simulink model "Distribution_vAggregate"  (Simulink 7.9)
settings: Solver=VariableStepDiscrete  StartTime=0.0  StopTime=1000  RelTol=1e-3
libraries: simeventslib x23
(part 3 of 4)

== system Distribution_vAggregate/Transportation_Channel_41 ==
  note: RESOURCE1 OUTBOUND
      | RESOURCE2 INBOUND
  note: RESOURCE1 INBOUND
      | RESOURCE2 OUTBOUND
  Enabled Gate : EnabledGate
  Enabled Gate1 : EnabledGate
  FIFO Queue : FIFOQueue  Capacity=inf  StatNumberInBlock=on
      settings: OutputPortMap=o1
  FIFO Queue1 : FIFOQueue  Capacity=inf  StatNumberInBlock=on
      settings: OutputPortMap=o1
  Inbound_Process_1 : InfiniteServer  ServiceTimeFrom=Signal port t  ServiceTime=(76.7)/30  StatNumberDeparted=on  StatNumberInBlock=on
      settings: OutputPortMap=o0,o1
  Inbound_Process_2 : InfiniteServer  ServiceTimeFrom=Signal port t  ServiceTime=(76.7)/30  StatNumberDeparted=on  StatNumberInBlock=on
      settings: OutputPortMap=o0,o1
  Inbound_Release_1 : SingleServer  ServiceTime=0  StatNumberInBlock=on
      settings: OutputPortMap=o1
  Inbound_Release_2 : SingleServer  ServiceTime=0  StatNumberInBlock=on
      settings: OutputPortMap=o1
  Infinite Server : InfiniteServer  ServiceTimeFrom=Signal port t  ServiceTime=(76.7)/30
  Infinite Server1 : InfiniteServer  ServiceTimeFrom=Signal port t  ServiceTime=(76.7)/30
  Mux : Mux  Inputs=3
  Outbound_Process_1 : InfiniteServer  ServiceTimeFrom=Signal port t  ServiceTime=(76.7)/30  StatNumberInBlock=on
      settings: OutputPortMap=o1
  Outbound_Process_2 : InfiniteServer  ServiceTimeFrom=Signal port t  ServiceTime=(76.7)/30  StatNumberInBlock=on
      settings: OutputPortMap=o1
  Outbound_Release_1 : SingleServer  ServiceTime=0  StatNumberInBlock=on
      settings: OutputPortMap=o1
  Outbound_Release_2 : SingleServer  ServiceTime=0  StatNumberInBlock=on
      settings: OutputPortMap=o1
  Sum{,1..2,4} (4 alike) : Sum  Inputs=|++
  Sum3 : Sum  Inputs=|++++
  TC_Status : simeventslib/SimEvents Sinks/Discrete Event Signal to Workspace  VariableName=Transportation_Channel_41_Status  SaveFormat=Structure With Time  isMonitorOnly=off  isRecordIC=off
  Timed to Event Signal : TimedToEventSignal
  TravelTime : Constant  Value=95.8472/30
  IN_Shipment_1 : PMIOPort  Port=1  Side=Left
  OUT_Shipment_1 : PMIOPort  Port=2  Side=Right
  IN_Resource_1 : PMIOPort  Port=3  Side=Left
  OUT_Resource_1 : PMIOPort  Port=4  Side=Right
  IN_Shipment_2 : PMIOPort  Port=5  Side=Left
  OUT_Shipment_2 : PMIOPort  Port=6  Side=Right
  IN_Resource_2 : PMIOPort  Port=7  Side=Left
  OUT_Resource_2 : PMIOPort  Port=8  Side=Right
  tag scope: Transportation_Channel_41_Status=global
  wires:
  Sum4/1 -> Mux/3
  Inbound_Process_2/1 -> Sum4/2
  Inbound_Process_1/1 -> Sum4/1
  Inbound_Process_2/2 -> Sum3/4
  Outbound_Process_2/1 -> Sum3/3
  Inbound_Process_1/2 -> Sum3/2
  Outbound_Process_1/1 -> Sum3/1
  Sum3/1 -> Mux/2
  Sum/1 -> Mux/1
  Mux/1 -> TC_Status/1, [Transportation_Channel_41_Status]
  Inbound_Release_2/1 -> Sum2/2
  Outbound_Release_1/1 -> Sum2/1
  Sum2/1 -> Enabled Gate/1
  Inbound_Release_1/1 -> Sum1/1
  Outbound_Release_2/1 -> Sum1/2
  Sum1/1 -> Enabled Gate1/1
  Timed to Event Signal/1 -> Infinite Server/1, Inbound_Process_2/1, Inbound_Process_1/1, Infinite Server1/1, Outbound_Process_2/1, Outbound_Process_1/1
  TravelTime/1 -> Timed to Event Signal/1
  FIFO Queue/1 -> Sum/1
  FIFO Queue1/1 -> Sum/2
  connections:
  Inbound_Process_1/RConn1 -- OUT_Resource_1/RConn1
  Outbound_Process_1/RConn1 -- Inbound_Release_1/LConn1
  Inbound_Release_1/RConn1 -- Inbound_Process_1/LConn1
  Outbound_Release_1/RConn1 -- Outbound_Process_1/LConn1
  Inbound_Process_2/RConn1 -- OUT_Resource_2/RConn1
  Inbound_Release_2/RConn1 -- Inbound_Process_2/LConn1
  Outbound_Process_2/RConn1 -- Inbound_Release_2/LConn1
  Outbound_Release_2/RConn1 -- Outbound_Process_2/LConn1
  IN_Resource_2/RConn1 -- Outbound_Release_2/LConn1
  Infinite Server1/RConn1 -- OUT_Shipment_1/RConn1
  Enabled Gate/RConn1 -- Infinite Server1/LConn1
  Infinite Server/LConn1 -- Enabled Gate1/RConn1
  OUT_Shipment_2/RConn1 -- Infinite Server/RConn1
  IN_Resource_1/RConn1 -- Outbound_Release_1/LConn1
  IN_Shipment_2/RConn1 -- FIFO Queue1/LConn1
  IN_Shipment_1/RConn1 -- FIFO Queue/LConn1
  Enabled Gate1/LConn1 -- FIFO Queue1/RConn1
  FIFO Queue/RConn1 -- Enabled Gate/LConn1

== system Distribution_vAggregate/Transportation_Channel_42 ==
  note: RESOURCE1 OUTBOUND
      | RESOURCE2 INBOUND
  note: RESOURCE1 INBOUND
      | RESOURCE2 OUTBOUND
  Enabled Gate : EnabledGate
  Enabled Gate1 : EnabledGate
  FIFO Queue : FIFOQueue  Capacity=inf  StatNumberInBlock=on
      settings: OutputPortMap=o1
  FIFO Queue1 : FIFOQueue  Capacity=inf  StatNumberInBlock=on
      settings: OutputPortMap=o1
  Inbound_Process_1 : InfiniteServer  ServiceTimeFrom=Signal port t  ServiceTime=(76.7)/30  StatNumberDeparted=on  StatNumberInBlock=on
      settings: OutputPortMap=o0,o1
  Inbound_Process_2 : InfiniteServer  ServiceTimeFrom=Signal port t  ServiceTime=(76.7)/30  StatNumberDeparted=on  StatNumberInBlock=on
      settings: OutputPortMap=o0,o1
  Inbound_Release_1 : SingleServer  ServiceTime=0  StatNumberInBlock=on
      settings: OutputPortMap=o1
  Inbound_Release_2 : SingleServer  ServiceTime=0  StatNumberInBlock=on
      settings: OutputPortMap=o1
  Infinite Server : InfiniteServer  ServiceTimeFrom=Signal port t  ServiceTime=(76.7)/30
  Infinite Server1 : InfiniteServer  ServiceTimeFrom=Signal port t  ServiceTime=(76.7)/30
  Mux : Mux  Inputs=3
  Outbound_Process_1 : InfiniteServer  ServiceTimeFrom=Signal port t  ServiceTime=(76.7)/30  StatNumberInBlock=on
      settings: OutputPortMap=o1
  Outbound_Process_2 : InfiniteServer  ServiceTimeFrom=Signal port t  ServiceTime=(76.7)/30  StatNumberInBlock=on
      settings: OutputPortMap=o1
  Outbound_Release_1 : SingleServer  ServiceTime=0  StatNumberInBlock=on
      settings: OutputPortMap=o1
  Outbound_Release_2 : SingleServer  ServiceTime=0  StatNumberInBlock=on
      settings: OutputPortMap=o1
  Sum{,1..2,4} (4 alike) : Sum  Inputs=|++
  Sum3 : Sum  Inputs=|++++
  TC_Status : simeventslib/SimEvents Sinks/Discrete Event Signal to Workspace  VariableName=Transportation_Channel_42_Status  SaveFormat=Structure With Time  isMonitorOnly=off  isRecordIC=off
  Timed to Event Signal : TimedToEventSignal
  TravelTime : Constant  Value=37.8123/30
  IN_Shipment_1 : PMIOPort  Port=1  Side=Left
  OUT_Shipment_1 : PMIOPort  Port=2  Side=Right
  IN_Resource_1 : PMIOPort  Port=3  Side=Left
  OUT_Resource_1 : PMIOPort  Port=4  Side=Right
  IN_Shipment_2 : PMIOPort  Port=5  Side=Left
  OUT_Shipment_2 : PMIOPort  Port=6  Side=Right
  IN_Resource_2 : PMIOPort  Port=7  Side=Left
  OUT_Resource_2 : PMIOPort  Port=8  Side=Right
  tag scope: Transportation_Channel_42_Status=global
  wires:
  Sum4/1 -> Mux/3
  Inbound_Process_2/1 -> Sum4/2
  Inbound_Process_1/1 -> Sum4/1
  Inbound_Process_2/2 -> Sum3/4
  Outbound_Process_2/1 -> Sum3/3
  Inbound_Process_1/2 -> Sum3/2
  Outbound_Process_1/1 -> Sum3/1
  Sum3/1 -> Mux/2
  Sum/1 -> Mux/1
  Mux/1 -> TC_Status/1, [Transportation_Channel_42_Status]
  Inbound_Release_2/1 -> Sum2/2
  Outbound_Release_1/1 -> Sum2/1
  Sum2/1 -> Enabled Gate/1
  Inbound_Release_1/1 -> Sum1/1
  Outbound_Release_2/1 -> Sum1/2
  Sum1/1 -> Enabled Gate1/1
  Timed to Event Signal/1 -> Infinite Server/1, Inbound_Process_2/1, Inbound_Process_1/1, Infinite Server1/1, Outbound_Process_2/1, Outbound_Process_1/1
  TravelTime/1 -> Timed to Event Signal/1
  FIFO Queue/1 -> Sum/1
  FIFO Queue1/1 -> Sum/2
  connections:
  Inbound_Process_1/RConn1 -- OUT_Resource_1/RConn1
  Outbound_Process_1/RConn1 -- Inbound_Release_1/LConn1
  Inbound_Release_1/RConn1 -- Inbound_Process_1/LConn1
  Outbound_Release_1/RConn1 -- Outbound_Process_1/LConn1
  Inbound_Process_2/RConn1 -- OUT_Resource_2/RConn1
  Inbound_Release_2/RConn1 -- Inbound_Process_2/LConn1
  Outbound_Process_2/RConn1 -- Inbound_Release_2/LConn1
  Outbound_Release_2/RConn1 -- Outbound_Process_2/LConn1
  IN_Resource_2/RConn1 -- Outbound_Release_2/LConn1
  Infinite Server1/RConn1 -- OUT_Shipment_1/RConn1
  Enabled Gate/RConn1 -- Infinite Server1/LConn1
  Infinite Server/LConn1 -- Enabled Gate1/RConn1
  OUT_Shipment_2/RConn1 -- Infinite Server/RConn1
  IN_Resource_1/RConn1 -- Outbound_Release_1/LConn1
  IN_Shipment_2/RConn1 -- FIFO Queue1/LConn1
  IN_Shipment_1/RConn1 -- FIFO Queue/LConn1
  Enabled Gate1/LConn1 -- FIFO Queue1/RConn1
  FIFO Queue/RConn1 -- Enabled Gate/LConn1

== system Distribution_vAggregate/Transportation_Channel_43 ==
  note: RESOURCE1 OUTBOUND
      | RESOURCE2 INBOUND
  note: RESOURCE1 INBOUND
      | RESOURCE2 OUTBOUND
  Enabled Gate : EnabledGate
  Enabled Gate1 : EnabledGate
  FIFO Queue : FIFOQueue  Capacity=inf  StatNumberInBlock=on
      settings: OutputPortMap=o1
  FIFO Queue1 : FIFOQueue  Capacity=inf  StatNumberInBlock=on
      settings: OutputPortMap=o1
  Inbound_Process_1 : InfiniteServer  ServiceTimeFrom=Signal port t  ServiceTime=(76.7)/30  StatNumberDeparted=on  StatNumberInBlock=on
      settings: OutputPortMap=o0,o1
  Inbound_Process_2 : InfiniteServer  ServiceTimeFrom=Signal port t  ServiceTime=(76.7)/30  StatNumberDeparted=on  StatNumberInBlock=on
      settings: OutputPortMap=o0,o1
  Inbound_Release_1 : SingleServer  ServiceTime=0  StatNumberInBlock=on
      settings: OutputPortMap=o1
  Inbound_Release_2 : SingleServer  ServiceTime=0  StatNumberInBlock=on
      settings: OutputPortMap=o1
  Infinite Server : InfiniteServer  ServiceTimeFrom=Signal port t  ServiceTime=(76.7)/30
  Infinite Server1 : InfiniteServer  ServiceTimeFrom=Signal port t  ServiceTime=(76.7)/30
  Mux : Mux  Inputs=3
  Outbound_Process_1 : InfiniteServer  ServiceTimeFrom=Signal port t  ServiceTime=(76.7)/30  StatNumberInBlock=on
      settings: OutputPortMap=o1
  Outbound_Process_2 : InfiniteServer  ServiceTimeFrom=Signal port t  ServiceTime=(76.7)/30  StatNumberInBlock=on
      settings: OutputPortMap=o1
  Outbound_Release_1 : SingleServer  ServiceTime=0  StatNumberInBlock=on
      settings: OutputPortMap=o1
  Outbound_Release_2 : SingleServer  ServiceTime=0  StatNumberInBlock=on
      settings: OutputPortMap=o1
  Sum{,1..2,4} (4 alike) : Sum  Inputs=|++
  Sum3 : Sum  Inputs=|++++
  TC_Status : simeventslib/SimEvents Sinks/Discrete Event Signal to Workspace  VariableName=Transportation_Channel_43_Status  SaveFormat=Structure With Time  isMonitorOnly=off  isRecordIC=off
  Timed to Event Signal : TimedToEventSignal
  TravelTime : Constant  Value=75.8703/30
  IN_Shipment_1 : PMIOPort  Port=1  Side=Left
  OUT_Shipment_1 : PMIOPort  Port=2  Side=Right
  IN_Resource_1 : PMIOPort  Port=3  Side=Left
  OUT_Resource_1 : PMIOPort  Port=4  Side=Right
  IN_Shipment_2 : PMIOPort  Port=5  Side=Left
  OUT_Shipment_2 : PMIOPort  Port=6  Side=Right
  IN_Resource_2 : PMIOPort  Port=7  Side=Left
  OUT_Resource_2 : PMIOPort  Port=8  Side=Right
  tag scope: Transportation_Channel_43_Status=global
  wires:
  Sum4/1 -> Mux/3
  Inbound_Process_2/1 -> Sum4/2
  Inbound_Process_1/1 -> Sum4/1
  Inbound_Process_2/2 -> Sum3/4
  Outbound_Process_2/1 -> Sum3/3
  Inbound_Process_1/2 -> Sum3/2
  Outbound_Process_1/1 -> Sum3/1
  Sum3/1 -> Mux/2
  Sum/1 -> Mux/1
  Mux/1 -> TC_Status/1, [Transportation_Channel_43_Status]
  Inbound_Release_2/1 -> Sum2/2
  Outbound_Release_1/1 -> Sum2/1
  Sum2/1 -> Enabled Gate/1
  Inbound_Release_1/1 -> Sum1/1
  Outbound_Release_2/1 -> Sum1/2
  Sum1/1 -> Enabled Gate1/1
  Timed to Event Signal/1 -> Infinite Server/1, Inbound_Process_2/1, Inbound_Process_1/1, Infinite Server1/1, Outbound_Process_2/1, Outbound_Process_1/1
  TravelTime/1 -> Timed to Event Signal/1
  FIFO Queue/1 -> Sum/1
  FIFO Queue1/1 -> Sum/2
  connections:
  Inbound_Process_1/RConn1 -- OUT_Resource_1/RConn1
  Outbound_Process_1/RConn1 -- Inbound_Release_1/LConn1
  Inbound_Release_1/RConn1 -- Inbound_Process_1/LConn1
  Outbound_Release_1/RConn1 -- Outbound_Process_1/LConn1
  Inbound_Process_2/RConn1 -- OUT_Resource_2/RConn1
  Inbound_Release_2/RConn1 -- Inbound_Process_2/LConn1
  Outbound_Process_2/RConn1 -- Inbound_Release_2/LConn1
  Outbound_Release_2/RConn1 -- Outbound_Process_2/LConn1
  IN_Resource_2/RConn1 -- Outbound_Release_2/LConn1
  Infinite Server1/RConn1 -- OUT_Shipment_1/RConn1
  Enabled Gate/RConn1 -- Infinite Server1/LConn1
  Infinite Server/LConn1 -- Enabled Gate1/RConn1
  OUT_Shipment_2/RConn1 -- Infinite Server/RConn1
  IN_Resource_1/RConn1 -- Outbound_Release_1/LConn1
  IN_Shipment_2/RConn1 -- FIFO Queue1/LConn1
  IN_Shipment_1/RConn1 -- FIFO Queue/LConn1
  Enabled Gate1/LConn1 -- FIFO Queue1/RConn1
  FIFO Queue/RConn1 -- Enabled Gate/LConn1

== system Distribution_vAggregate/Customer_1/Commodity_1 ==
  Clock : Clock
  Source : TimeBasedEntityGenerator  Distribution=Exponential  InitialSeed=7493  Mean=Mean  GenerateEntityAtSimulationStart=off
  Timed to Event Signal : TimedToEventSignal
  setAttribute : SetAttribute  AttributeName=Route|Origin|Destination|Start  AttributeFrom=Dialog|Dialog|Dialog|Signal port  AttributeValue="[1  17  15   2   0   0]|1|2|1"  AttributeTreatAsVector=0|1|1|1  EvaluatedAttributeValue="{[1  17  15   2   0   0];1;2;[]}"
      settings: InputPortMap=u3
  OUT_Commodity : PMIOPort  Port=1  Side=Right
  wires:
  Timed to Event Signal/1 -> setAttribute/1
  Clock/1 -> Timed to Event Signal/1
  connections:
  OUT_Commodity/RConn1 -- setAttribute/RConn1
  Source/RConn1 -- setAttribute/LConn1

== system Distribution_vAggregate/Customer_1/Commodity_2 ==
  Clock : Clock
  Source : TimeBasedEntityGenerator  Distribution=Exponential  InitialSeed=10710  Mean=Mean  GenerateEntityAtSimulationStart=off
  Timed to Event Signal : TimedToEventSignal
  setAttribute : SetAttribute  AttributeName=Route|Origin|Destination|Start  AttributeFrom=Dialog|Dialog|Dialog|Signal port  AttributeValue="[1  17  15   3   0   0]|1|3|1"  AttributeTreatAsVector=0|1|1|1  EvaluatedAttributeValue="{[1  17  15   3   0   0];1;3;[]}"
      settings: InputPortMap=u3
  OUT_Commodity : PMIOPort  Port=1  Side=Right
  wires:
  Timed to Event Signal/1 -> setAttribute/1
  Clock/1 -> Timed to Event Signal/1
  connections:
  OUT_Commodity/RConn1 -- setAttribute/RConn1
  Source/RConn1 -- setAttribute/LConn1

== system Distribution_vAggregate/Customer_1/Commodity_3 ==
  Clock : Clock
  Source : TimeBasedEntityGenerator  Distribution=Exponential  InitialSeed=13927  Mean=Mean  GenerateEntityAtSimulationStart=off
  Timed to Event Signal : TimedToEventSignal
  setAttribute : SetAttribute  AttributeName=Route|Origin|Destination|Start  AttributeFrom=Dialog|Dialog|Dialog|Signal port  AttributeValue="[1  17  12   4   0   0]|1|4|1"  AttributeTreatAsVector=0|1|1|1  EvaluatedAttributeValue="{[1  17  12   4   0   0];1;4;[]}"
      settings: InputPortMap=u3
  OUT_Commodity : PMIOPort  Port=1  Side=Right
  wires:
  Timed to Event Signal/1 -> setAttribute/1
  Clock/1 -> Timed to Event Signal/1
  connections:
  OUT_Commodity/RConn1 -- setAttribute/RConn1
  Source/RConn1 -- setAttribute/LConn1

== system Distribution_vAggregate/Customer_1/Commodity_4 ==
  Clock : Clock
  Source : TimeBasedEntityGenerator  Distribution=Exponential  InitialSeed=17144  Mean=Mean  GenerateEntityAtSimulationStart=off
  Timed to Event Signal : TimedToEventSignal
  setAttribute : SetAttribute  AttributeName=Route|Origin|Destination|Start  AttributeFrom=Dialog|Dialog|Dialog|Signal port  AttributeValue="[1  17  12   5   0   0]|1|5|1"  AttributeTreatAsVector=0|1|1|1  EvaluatedAttributeValue="{[1  17  12   5   0   0];1;5;[]}"
      settings: InputPortMap=u3
  OUT_Commodity : PMIOPort  Port=1  Side=Right
  wires:
  Timed to Event Signal/1 -> setAttribute/1
  Clock/1 -> Timed to Event Signal/1
  connections:
  OUT_Commodity/RConn1 -- setAttribute/RConn1
  Source/RConn1 -- setAttribute/LConn1

== system Distribution_vAggregate/Customer_1/Commodity_5 ==
  Clock : Clock
  Source : TimeBasedEntityGenerator  Distribution=Exponential  InitialSeed=20361  Mean=Mean  GenerateEntityAtSimulationStart=off
  Timed to Event Signal : TimedToEventSignal
  setAttribute : SetAttribute  AttributeName=Route|Origin|Destination|Start  AttributeFrom=Dialog|Dialog|Dialog|Signal port  AttributeValue="[1  17  12   6   0   0]|1|6|1"  AttributeTreatAsVector=0|1|1|1  EvaluatedAttributeValue="{[1  17  12   6   0   0];1;6;[]}"
      settings: InputPortMap=u3
  OUT_Commodity : PMIOPort  Port=1  Side=Right
  wires:
  Timed to Event Signal/1 -> setAttribute/1
  Clock/1 -> Timed to Event Signal/1
  connections:
  OUT_Commodity/RConn1 -- setAttribute/RConn1
  Source/RConn1 -- setAttribute/LConn1

== system Distribution_vAggregate/Customer_1/Commodity_6 ==
  Clock : Clock
  Source : TimeBasedEntityGenerator  Distribution=Exponential  InitialSeed=23578  Mean=Mean  GenerateEntityAtSimulationStart=off
  Timed to Event Signal : TimedToEventSignal
  setAttribute : SetAttribute  AttributeName=Route|Origin|Destination|Start  AttributeFrom=Dialog|Dialog|Dialog|Signal port  AttributeValue="[1  17  12   7   0   0]|1|7|1"  AttributeTreatAsVector=0|1|1|1  EvaluatedAttributeValue="{[1  17  12   7   0   0];1;7;[]}"
      settings: InputPortMap=u3
  OUT_Commodity : PMIOPort  Port=1  Side=Right
  wires:
  Timed to Event Signal/1 -> setAttribute/1
  Clock/1 -> Timed to Event Signal/1
  connections:
  OUT_Commodity/RConn1 -- setAttribute/RConn1
  Source/RConn1 -- setAttribute/LConn1

== system Distribution_vAggregate/Customer_1/Commodity_7 ==
  Clock : Clock
  Source : TimeBasedEntityGenerator  Distribution=Exponential  InitialSeed=26795  Mean=Mean  GenerateEntityAtSimulationStart=off
  Timed to Event Signal : TimedToEventSignal
  setAttribute : SetAttribute  AttributeName=Route|Origin|Destination|Start  AttributeFrom=Dialog|Dialog|Dialog|Signal port  AttributeValue="[1  17  15   8   0   0]|1|8|1"  AttributeTreatAsVector=0|1|1|1  EvaluatedAttributeValue="{[1  17  15   8   0   0];1;8;[]}"
      settings: InputPortMap=u3
  OUT_Commodity : PMIOPort  Port=1  Side=Right
  wires:
  Timed to Event Signal/1 -> setAttribute/1
  Clock/1 -> Timed to Event Signal/1
  connections:
  OUT_Commodity/RConn1 -- setAttribute/RConn1
  Source/RConn1 -- setAttribute/LConn1

== system Distribution_vAggregate/Customer_1/Commodity_8 ==
  Clock : Clock
  Source : TimeBasedEntityGenerator  Distribution=Exponential  InitialSeed=30012  Mean=Mean  GenerateEntityAtSimulationStart=off
  Timed to Event Signal : TimedToEventSignal
  setAttribute : SetAttribute  AttributeName=Route|Origin|Destination|Start  AttributeFrom=Dialog|Dialog|Dialog|Signal port  AttributeValue="[1  17  15   9   0   0]|1|9|1"  AttributeTreatAsVector=0|1|1|1  EvaluatedAttributeValue="{[1  17  15   9   0   0];1;9;[]}"
      settings: InputPortMap=u3
  OUT_Commodity : PMIOPort  Port=1  Side=Right
  wires:
  Timed to Event Signal/1 -> setAttribute/1
  Clock/1 -> Timed to Event Signal/1
  connections:
  OUT_Commodity/RConn1 -- setAttribute/RConn1
  Source/RConn1 -- setAttribute/LConn1

== system Distribution_vAggregate/Customer_1/Commodity_9 ==
  Clock : Clock
  Source : TimeBasedEntityGenerator  Distribution=Exponential  InitialSeed=33229  Mean=Mean  GenerateEntityAtSimulationStart=off
  Timed to Event Signal : TimedToEventSignal
  setAttribute : SetAttribute  AttributeName=Route|Origin|Destination|Start  AttributeFrom=Dialog|Dialog|Dialog|Signal port  AttributeValue="[1  17  12  10   0   0]|1|10|1"  AttributeTreatAsVector=0|1|1|1  EvaluatedAttributeValue="{[1  17  12  10   0   0];1;10;[]}"
      settings: InputPortMap=u3
  OUT_Commodity : PMIOPort  Port=1  Side=Right
  wires:
  Timed to Event Signal/1 -> setAttribute/1
  Clock/1 -> Timed to Event Signal/1
  connections:
  OUT_Commodity/RConn1 -- setAttribute/RConn1
  Source/RConn1 -- setAttribute/LConn1

== system Distribution_vAggregate/Customer_10/Commodity_82 ==
  Clock : Clock
  Source : TimeBasedEntityGenerator  Distribution=Exponential  InitialSeed=36446  Mean=Mean  GenerateEntityAtSimulationStart=off
  Timed to Event Signal : TimedToEventSignal
  setAttribute : SetAttribute  AttributeName=Route|Origin|Destination|Start  AttributeFrom=Dialog|Dialog|Dialog|Signal port  AttributeValue="[10  12  17   1   0   0]|10|1|1"  AttributeTreatAsVector=0|1|1|1  EvaluatedAttributeValue="{[10  12  17   1   0   0];10;1;[]}"
      settings: InputPortMap=u3
  OUT_Commodity : PMIOPort  Port=1  Side=Right
  wires:
  Timed to Event Signal/1 -> setAttribute/1
  Clock/1 -> Timed to Event Signal/1
  connections:
  OUT_Commodity/RConn1 -- setAttribute/RConn1
  Source/RConn1 -- setAttribute/LConn1

== system Distribution_vAggregate/Customer_10/Commodity_83 ==
  Clock : Clock
  Source : TimeBasedEntityGenerator  Distribution=Exponential  InitialSeed=39663  Mean=Mean  GenerateEntityAtSimulationStart=off
  Timed to Event Signal : TimedToEventSignal
  setAttribute : SetAttribute  AttributeName=Route|Origin|Destination|Start  AttributeFrom=Dialog|Dialog|Dialog|Signal port  AttributeValue="[10  12  15   2   0   0]|10|2|1"  AttributeTreatAsVector=0|1|1|1  EvaluatedAttributeValue="{[10  12  15   2   0   0];10;2;[]}"
      settings: InputPortMap=u3
  OUT_Commodity : PMIOPort  Port=1  Side=Right
  wires:
  Timed to Event Signal/1 -> setAttribute/1
  Clock/1 -> Timed to Event Signal/1
  connections:
  OUT_Commodity/RConn1 -- setAttribute/RConn1
  Source/RConn1 -- setAttribute/LConn1

== system Distribution_vAggregate/Customer_10/Commodity_84 ==
  Clock : Clock
  Source : TimeBasedEntityGenerator  Distribution=Exponential  InitialSeed=42880  Mean=Mean  GenerateEntityAtSimulationStart=off
  Timed to Event Signal : TimedToEventSignal
  setAttribute : SetAttribute  AttributeName=Route|Origin|Destination|Start  AttributeFrom=Dialog|Dialog|Dialog|Signal port  AttributeValue="[10  12  15   3   0   0]|10|3|1"  AttributeTreatAsVector=0|1|1|1  EvaluatedAttributeValue="{[10  12  15   3   0   0];10;3;[]}"
      settings: InputPortMap=u3
  OUT_Commodity : PMIOPort  Port=1  Side=Right
  wires:
  Timed to Event Signal/1 -> setAttribute/1
  Clock/1 -> Timed to Event Signal/1
  connections:
  OUT_Commodity/RConn1 -- setAttribute/RConn1
  Source/RConn1 -- setAttribute/LConn1

== system Distribution_vAggregate/Customer_10/Commodity_85 ==
  Clock : Clock
  Source : TimeBasedEntityGenerator  Distribution=Exponential  InitialSeed=46097  Mean=Mean  GenerateEntityAtSimulationStart=off
  Timed to Event Signal : TimedToEventSignal
  setAttribute : SetAttribute  AttributeName=Route|Origin|Destination|Start  AttributeFrom=Dialog|Dialog|Dialog|Signal port  AttributeValue="[10  12   4   0   0   0]|10|4|1"  AttributeTreatAsVector=0|1|1|1  EvaluatedAttributeValue="{[10  12   4   0   0   0];10;4;[]}"
      settings: InputPortMap=u3
  OUT_Commodity : PMIOPort  Port=1  Side=Right
  wires:
  Timed to Event Signal/1 -> setAttribute/1
  Clock/1 -> Timed to Event Signal/1
  connections:
  OUT_Commodity/RConn1 -- setAttribute/RConn1
  Source/RConn1 -- setAttribute/LConn1

== system Distribution_vAggregate/Customer_10/Commodity_86 ==
  Clock : Clock
  Source : TimeBasedEntityGenerator  Distribution=Exponential  InitialSeed=49314  Mean=Mean  GenerateEntityAtSimulationStart=off
  Timed to Event Signal : TimedToEventSignal
  setAttribute : SetAttribute  AttributeName=Route|Origin|Destination|Start  AttributeFrom=Dialog|Dialog|Dialog|Signal port  AttributeValue="[10  12   5   0   0   0]|10|5|1"  AttributeTreatAsVector=0|1|1|1  EvaluatedAttributeValue="{[10  12   5   0   0   0];10;5;[]}"
      settings: InputPortMap=u3
  OUT_Commodity : PMIOPort  Port=1  Side=Right
  wires:
  Timed to Event Signal/1 -> setAttribute/1
  Clock/1 -> Timed to Event Signal/1
  connections:
  OUT_Commodity/RConn1 -- setAttribute/RConn1
  Source/RConn1 -- setAttribute/LConn1

== system Distribution_vAggregate/Customer_10/Commodity_87 ==
  Clock : Clock
  Source : TimeBasedEntityGenerator  Distribution=Exponential  InitialSeed=52531  Mean=Mean  GenerateEntityAtSimulationStart=off
  Timed to Event Signal : TimedToEventSignal
  setAttribute : SetAttribute  AttributeName=Route|Origin|Destination|Start  AttributeFrom=Dialog|Dialog|Dialog|Signal port  AttributeValue="[10  12   6   0   0   0]|10|6|1"  AttributeTreatAsVector=0|1|1|1  EvaluatedAttributeValue="{[10  12   6   0   0   0];10;6;[]}"
      settings: InputPortMap=u3
  OUT_Commodity : PMIOPort  Port=1  Side=Right
  wires:
  Timed to Event Signal/1 -> setAttribute/1
  Clock/1 -> Timed to Event Signal/1
  connections:
  OUT_Commodity/RConn1 -- setAttribute/RConn1
  Source/RConn1 -- setAttribute/LConn1

== system Distribution_vAggregate/Customer_10/Commodity_88 ==
  Clock : Clock
  Source : TimeBasedEntityGenerator  Distribution=Exponential  InitialSeed=55748  Mean=Mean  GenerateEntityAtSimulationStart=off
  Timed to Event Signal : TimedToEventSignal
  setAttribute : SetAttribute  AttributeName=Route|Origin|Destination|Start  AttributeFrom=Dialog|Dialog|Dialog|Signal port  AttributeValue="[10  12   7   0   0   0]|10|7|1"  AttributeTreatAsVector=0|1|1|1  EvaluatedAttributeValue="{[10  12   7   0   0   0];10;7;[]}"
      settings: InputPortMap=u3
  OUT_Commodity : PMIOPort  Port=1  Side=Right
  wires:
  Timed to Event Signal/1 -> setAttribute/1
  Clock/1 -> Timed to Event Signal/1
  connections:
  OUT_Commodity/RConn1 -- setAttribute/RConn1
  Source/RConn1 -- setAttribute/LConn1

== system Distribution_vAggregate/Customer_10/Commodity_89 ==
  Clock : Clock
  Source : TimeBasedEntityGenerator  Distribution=Exponential  InitialSeed=58965  Mean=Mean  GenerateEntityAtSimulationStart=off
  Timed to Event Signal : TimedToEventSignal
  setAttribute : SetAttribute  AttributeName=Route|Origin|Destination|Start  AttributeFrom=Dialog|Dialog|Dialog|Signal port  AttributeValue="[10  12  15   8   0   0]|10|8|1"  AttributeTreatAsVector=0|1|1|1  EvaluatedAttributeValue="{[10  12  15   8   0   0];10;8;[]}"
      settings: InputPortMap=u3
  OUT_Commodity : PMIOPort  Port=1  Side=Right
  wires:
  Timed to Event Signal/1 -> setAttribute/1
  Clock/1 -> Timed to Event Signal/1
  connections:
  OUT_Commodity/RConn1 -- setAttribute/RConn1
  Source/RConn1 -- setAttribute/LConn1

== system Distribution_vAggregate/Customer_10/Commodity_90 ==
  Clock : Clock
  Source : TimeBasedEntityGenerator  Distribution=Exponential  InitialSeed=62182  Mean=Mean  GenerateEntityAtSimulationStart=off
  Timed to Event Signal : TimedToEventSignal
  setAttribute : SetAttribute  AttributeName=Route|Origin|Destination|Start  AttributeFrom=Dialog|Dialog|Dialog|Signal port  AttributeValue="[10  12  15   9   0   0]|10|9|1"  AttributeTreatAsVector=0|1|1|1  EvaluatedAttributeValue="{[10  12  15   9   0   0];10;9;[]}"
      settings: InputPortMap=u3
  OUT_Commodity : PMIOPort  Port=1  Side=Right
  wires:
  Timed to Event Signal/1 -> setAttribute/1
  Clock/1 -> Timed to Event Signal/1
  connections:
  OUT_Commodity/RConn1 -- setAttribute/RConn1
  Source/RConn1 -- setAttribute/LConn1

== system Distribution_vAggregate/Customer_2/Commodity_10 ==
  Clock : Clock
  Source : TimeBasedEntityGenerator  Distribution=Exponential  InitialSeed=65399  Mean=Mean  GenerateEntityAtSimulationStart=off
  Timed to Event Signal : TimedToEventSignal
  setAttribute : SetAttribute  AttributeName=Route|Origin|Destination|Start  AttributeFrom=Dialog|Dialog|Dialog|Signal port  AttributeValue="[2  15  17   1   0   0]|2|1|1"  AttributeTreatAsVector=0|1|1|1  EvaluatedAttributeValue="{[2  15  17   1   0   0];2;1;[]}"
      settings: InputPortMap=u3
  OUT_Commodity : PMIOPort  Port=1  Side=Right
  wires:
  Timed to Event Signal/1 -> setAttribute/1
  Clock/1 -> Timed to Event Signal/1
  connections:
  OUT_Commodity/RConn1 -- setAttribute/RConn1
  Source/RConn1 -- setAttribute/LConn1

== system Distribution_vAggregate/Customer_2/Commodity_11 ==
  Clock : Clock
  Source : TimeBasedEntityGenerator  Distribution=Exponential  InitialSeed=3080  Mean=Mean  GenerateEntityAtSimulationStart=off
  Timed to Event Signal : TimedToEventSignal
  setAttribute : SetAttribute  AttributeName=Route|Origin|Destination|Start  AttributeFrom=Dialog|Dialog|Dialog|Signal port  AttributeValue="[2  15   3   0   0   0]|2|3|1"  AttributeTreatAsVector=0|1|1|1  EvaluatedAttributeValue="{[2  15   3   0   0   0];2;3;[]}"
      settings: InputPortMap=u3
  OUT_Commodity : PMIOPort  Port=1  Side=Right
  wires:
  Timed to Event Signal/1 -> setAttribute/1
  Clock/1 -> Timed to Event Signal/1
  connections:
  OUT_Commodity/RConn1 -- setAttribute/RConn1
  Source/RConn1 -- setAttribute/LConn1

== system Distribution_vAggregate/Customer_2/Commodity_12 ==
  Clock : Clock
  Source : TimeBasedEntityGenerator  Distribution=Exponential  InitialSeed=6297  Mean=Mean  GenerateEntityAtSimulationStart=off
  Timed to Event Signal : TimedToEventSignal
  setAttribute : SetAttribute  AttributeName=Route|Origin|Destination|Start  AttributeFrom=Dialog|Dialog|Dialog|Signal port  AttributeValue="[2  15  12   4   0   0]|2|4|1"  AttributeTreatAsVector=0|1|1|1  EvaluatedAttributeValue="{[2  15  12   4   0   0];2;4;[]}"
      settings: InputPortMap=u3
  OUT_Commodity : PMIOPort  Port=1  Side=Right
  wires:
  Timed to Event Signal/1 -> setAttribute/1
  Clock/1 -> Timed to Event Signal/1
  connections:
  OUT_Commodity/RConn1 -- setAttribute/RConn1
  Source/RConn1 -- setAttribute/LConn1

== system Distribution_vAggregate/Customer_2/Commodity_13 ==
  Clock : Clock
  Source : TimeBasedEntityGenerator  Distribution=Exponential  InitialSeed=9514  Mean=Mean  GenerateEntityAtSimulationStart=off
  Timed to Event Signal : TimedToEventSignal
  setAttribute : SetAttribute  AttributeName=Route|Origin|Destination|Start  AttributeFrom=Dialog|Dialog|Dialog|Signal port  AttributeValue="[2  15  12   5   0   0]|2|5|1"  AttributeTreatAsVector=0|1|1|1  EvaluatedAttributeValue="{[2  15  12   5   0   0];2;5;[]}"
      settings: InputPortMap=u3
  OUT_Commodity : PMIOPort  Port=1  Side=Right
  wires:
  Timed to Event Signal/1 -> setAttribute/1
  Clock/1 -> Timed to Event Signal/1
  connections:
  OUT_Commodity/RConn1 -- setAttribute/RConn1
  Source/RConn1 -- setAttribute/LConn1

== system Distribution_vAggregate/Customer_2/Commodity_14 ==
  Clock : Clock
  Source : TimeBasedEntityGenerator  Distribution=Exponential  InitialSeed=12731  Mean=Mean  GenerateEntityAtSimulationStart=off
  Timed to Event Signal : TimedToEventSignal
  setAttribute : SetAttribute  AttributeName=Route|Origin|Destination|Start  AttributeFrom=Dialog|Dialog|Dialog|Signal port  AttributeValue="[2  15  12   6   0   0]|2|6|1"  AttributeTreatAsVector=0|1|1|1  EvaluatedAttributeValue="{[2  15  12   6   0   0];2;6;[]}"
      settings: InputPortMap=u3
  OUT_Commodity : PMIOPort  Port=1  Side=Right
  wires:
  Timed to Event Signal/1 -> setAttribute/1
  Clock/1 -> Timed to Event Signal/1
  connections:
  OUT_Commodity/RConn1 -- setAttribute/RConn1
  Source/RConn1 -- setAttribute/LConn1

== system Distribution_vAggregate/Customer_2/Commodity_15 ==
  Clock : Clock
  Source : TimeBasedEntityGenerator  Distribution=Exponential  InitialSeed=15948  Mean=Mean  GenerateEntityAtSimulationStart=off
  Timed to Event Signal : TimedToEventSignal
  setAttribute : SetAttribute  AttributeName=Route|Origin|Destination|Start  AttributeFrom=Dialog|Dialog|Dialog|Signal port  AttributeValue="[2  15  12   7   0   0]|2|7|1"  AttributeTreatAsVector=0|1|1|1  EvaluatedAttributeValue="{[2  15  12   7   0   0];2;7;[]}"
      settings: InputPortMap=u3
  OUT_Commodity : PMIOPort  Port=1  Side=Right
  wires:
  Timed to Event Signal/1 -> setAttribute/1
  Clock/1 -> Timed to Event Signal/1
  connections:
  OUT_Commodity/RConn1 -- setAttribute/RConn1
  Source/RConn1 -- setAttribute/LConn1

== system Distribution_vAggregate/Customer_2/Commodity_16 ==
  Clock : Clock
  Source : TimeBasedEntityGenerator  Distribution=Exponential  InitialSeed=19165  Mean=Mean  GenerateEntityAtSimulationStart=off
  Timed to Event Signal : TimedToEventSignal
  setAttribute : SetAttribute  AttributeName=Route|Origin|Destination|Start  AttributeFrom=Dialog|Dialog|Dialog|Signal port  AttributeValue="[2  15   8   0   0   0]|2|8|1"  AttributeTreatAsVector=0|1|1|1  EvaluatedAttributeValue="{[2  15   8   0   0   0];2;8;[]}"
      settings: InputPortMap=u3
  OUT_Commodity : PMIOPort  Port=1  Side=Right
  wires:
  Timed to Event Signal/1 -> setAttribute/1
  Clock/1 -> Timed to Event Signal/1
  connections:
  OUT_Commodity/RConn1 -- setAttribute/RConn1
  Source/RConn1 -- setAttribute/LConn1

== system Distribution_vAggregate/Customer_2/Commodity_17 ==
  Clock : Clock
  Source : TimeBasedEntityGenerator  Distribution=Exponential  InitialSeed=22382  Mean=Mean  GenerateEntityAtSimulationStart=off
  Timed to Event Signal : TimedToEventSignal
  setAttribute : SetAttribute  AttributeName=Route|Origin|Destination|Start  AttributeFrom=Dialog|Dialog|Dialog|Signal port  AttributeValue="[2  15   9   0   0   0]|2|9|1"  AttributeTreatAsVector=0|1|1|1  EvaluatedAttributeValue="{[2  15   9   0   0   0];2;9;[]}"
      settings: InputPortMap=u3
  OUT_Commodity : PMIOPort  Port=1  Side=Right
  wires:
  Timed to Event Signal/1 -> setAttribute/1
  Clock/1 -> Timed to Event Signal/1
  connections:
  OUT_Commodity/RConn1 -- setAttribute/RConn1
  Source/RConn1 -- setAttribute/LConn1

== system Distribution_vAggregate/Customer_2/Commodity_18 ==
  Clock : Clock
  Source : TimeBasedEntityGenerator  Distribution=Exponential  InitialSeed=25599  Mean=Mean  GenerateEntityAtSimulationStart=off
  Timed to Event Signal : TimedToEventSignal
  setAttribute : SetAttribute  AttributeName=Route|Origin|Destination|Start  AttributeFrom=Dialog|Dialog|Dialog|Signal port  AttributeValue="[2  15  12  10   0   0]|2|10|1"  AttributeTreatAsVector=0|1|1|1  EvaluatedAttributeValue="{[2  15  12  10   0   0];2;10;[]}"
      settings: InputPortMap=u3
  OUT_Commodity : PMIOPort  Port=1  Side=Right
  wires:
  Timed to Event Signal/1 -> setAttribute/1
  Clock/1 -> Timed to Event Signal/1
  connections:
  OUT_Commodity/RConn1 -- setAttribute/RConn1
  Source/RConn1 -- setAttribute/LConn1

== system Distribution_vAggregate/Customer_3/Commodity_19 ==
  Clock : Clock
  Source : TimeBasedEntityGenerator  Distribution=Exponential  InitialSeed=28816  Mean=Mean  GenerateEntityAtSimulationStart=off
  Timed to Event Signal : TimedToEventSignal
  setAttribute : SetAttribute  AttributeName=Route|Origin|Destination|Start  AttributeFrom=Dialog|Dialog|Dialog|Signal port  AttributeValue="[3  15  17   1   0   0]|3|1|1"  AttributeTreatAsVector=0|1|1|1  EvaluatedAttributeValue="{[3  15  17   1   0   0];3;1;[]}"
      settings: InputPortMap=u3
  OUT_Commodity : PMIOPort  Port=1  Side=Right
  wires:
  Timed to Event Signal/1 -> setAttribute/1
  Clock/1 -> Timed to Event Signal/1
  connections:
  OUT_Commodity/RConn1 -- setAttribute/RConn1
  Source/RConn1 -- setAttribute/LConn1

== system Distribution_vAggregate/Customer_3/Commodity_20 ==
  Clock : Clock
  Source : TimeBasedEntityGenerator  Distribution=Exponential  InitialSeed=32033  Mean=Mean  GenerateEntityAtSimulationStart=off
  Timed to Event Signal : TimedToEventSignal
  setAttribute : SetAttribute  AttributeName=Route|Origin|Destination|Start  AttributeFrom=Dialog|Dialog|Dialog|Signal port  AttributeValue="[3  15   2   0   0   0]|3|2|1"  AttributeTreatAsVector=0|1|1|1  EvaluatedAttributeValue="{[3  15   2   0   0   0];3;2;[]}"
      settings: InputPortMap=u3
  OUT_Commodity : PMIOPort  Port=1  Side=Right
  wires:
  Timed to Event Signal/1 -> setAttribute/1
  Clock/1 -> Timed to Event Signal/1
  connections:
  OUT_Commodity/RConn1 -- setAttribute/RConn1
  Source/RConn1 -- setAttribute/LConn1

== system Distribution_vAggregate/Customer_3/Commodity_21 ==
  Clock : Clock
  Source : TimeBasedEntityGenerator  Distribution=Exponential  InitialSeed=35250  Mean=Mean  GenerateEntityAtSimulationStart=off
  Timed to Event Signal : TimedToEventSignal
  setAttribute : SetAttribute  AttributeName=Route|Origin|Destination|Start  AttributeFrom=Dialog|Dialog|Dialog|Signal port  AttributeValue="[3  15  12   4   0   0]|3|4|1"  AttributeTreatAsVector=0|1|1|1  EvaluatedAttributeValue="{[3  15  12   4   0   0];3;4;[]}"
      settings: InputPortMap=u3
  OUT_Commodity : PMIOPort  Port=1  Side=Right
  wires:
  Timed to Event Signal/1 -> setAttribute/1
  Clock/1 -> Timed to Event Signal/1
  connections:
  OUT_Commodity/RConn1 -- setAttribute/RConn1
  Source/RConn1 -- setAttribute/LConn1

== system Distribution_vAggregate/Customer_3/Commodity_22 ==
  Clock : Clock
  Source : TimeBasedEntityGenerator  Distribution=Exponential  InitialSeed=38467  Mean=Mean  GenerateEntityAtSimulationStart=off
  Timed to Event Signal : TimedToEventSignal
  setAttribute : SetAttribute  AttributeName=Route|Origin|Destination|Start  AttributeFrom=Dialog|Dialog|Dialog|Signal port  AttributeValue="[3  15  12   5   0   0]|3|5|1"  AttributeTreatAsVector=0|1|1|1  EvaluatedAttributeValue="{[3  15  12   5   0   0];3;5;[]}"
      settings: InputPortMap=u3
  OUT_Commodity : PMIOPort  Port=1  Side=Right
  wires:
  Timed to Event Signal/1 -> setAttribute/1
  Clock/1 -> Timed to Event Signal/1
  connections:
  OUT_Commodity/RConn1 -- setAttribute/RConn1
  Source/RConn1 -- setAttribute/LConn1

== system Distribution_vAggregate/Customer_3/Commodity_23 ==
  Clock : Clock
  Source : TimeBasedEntityGenerator  Distribution=Exponential  InitialSeed=41684  Mean=Mean  GenerateEntityAtSimulationStart=off
  Timed to Event Signal : TimedToEventSignal
  setAttribute : SetAttribute  AttributeName=Route|Origin|Destination|Start  AttributeFrom=Dialog|Dialog|Dialog|Signal port  AttributeValue="[3  15  12   6   0   0]|3|6|1"  AttributeTreatAsVector=0|1|1|1  EvaluatedAttributeValue="{[3  15  12   6   0   0];3;6;[]}"
      settings: InputPortMap=u3
  OUT_Commodity : PMIOPort  Port=1  Side=Right
  wires:
  Timed to Event Signal/1 -> setAttribute/1
  Clock/1 -> Timed to Event Signal/1
  connections:
  OUT_Commodity/RConn1 -- setAttribute/RConn1
  Source/RConn1 -- setAttribute/LConn1

== system Distribution_vAggregate/Customer_3/Commodity_24 ==
  Clock : Clock
  Source : TimeBasedEntityGenerator  Distribution=Exponential  InitialSeed=44901  Mean=Mean  GenerateEntityAtSimulationStart=off
  Timed to Event Signal : TimedToEventSignal
  setAttribute : SetAttribute  AttributeName=Route|Origin|Destination|Start  AttributeFrom=Dialog|Dialog|Dialog|Signal port  AttributeValue="[3  15  12   7   0   0]|3|7|1"  AttributeTreatAsVector=0|1|1|1  EvaluatedAttributeValue="{[3  15  12   7   0   0];3;7;[]}"
      settings: InputPortMap=u3
  OUT_Commodity : PMIOPort  Port=1  Side=Right
  wires:
  Timed to Event Signal/1 -> setAttribute/1
  Clock/1 -> Timed to Event Signal/1
  connections:
  OUT_Commodity/RConn1 -- setAttribute/RConn1
  Source/RConn1 -- setAttribute/LConn1

== system Distribution_vAggregate/Customer_3/Commodity_25 ==
  Clock : Clock
  Source : TimeBasedEntityGenerator  Distribution=Exponential  InitialSeed=48118  Mean=Mean  GenerateEntityAtSimulationStart=off
  Timed to Event Signal : TimedToEventSignal
  setAttribute : SetAttribute  AttributeName=Route|Origin|Destination|Start  AttributeFrom=Dialog|Dialog|Dialog|Signal port  AttributeValue="[3  15   8   0   0   0]|3|8|1"  AttributeTreatAsVector=0|1|1|1  EvaluatedAttributeValue="{[3  15   8   0   0   0];3;8;[]}"
      settings: InputPortMap=u3
  OUT_Commodity : PMIOPort  Port=1  Side=Right
  wires:
  Timed to Event Signal/1 -> setAttribute/1
  Clock/1 -> Timed to Event Signal/1
  connections:
  OUT_Commodity/RConn1 -- setAttribute/RConn1
  Source/RConn1 -- setAttribute/LConn1

== system Distribution_vAggregate/Customer_3/Commodity_26 ==
  Clock : Clock
  Source : TimeBasedEntityGenerator  Distribution=Exponential  InitialSeed=51335  Mean=Mean  GenerateEntityAtSimulationStart=off
  Timed to Event Signal : TimedToEventSignal
  setAttribute : SetAttribute  AttributeName=Route|Origin|Destination|Start  AttributeFrom=Dialog|Dialog|Dialog|Signal port  AttributeValue="[3  15   9   0   0   0]|3|9|1"  AttributeTreatAsVector=0|1|1|1  EvaluatedAttributeValue="{[3  15   9   0   0   0];3;9;[]}"
      settings: InputPortMap=u3
  OUT_Commodity : PMIOPort  Port=1  Side=Right
  wires:
  Timed to Event Signal/1 -> setAttribute/1
  Clock/1 -> Timed to Event Signal/1
  connections:
  OUT_Commodity/RConn1 -- setAttribute/RConn1
  Source/RConn1 -- setAttribute/LConn1

== system Distribution_vAggregate/Customer_3/Commodity_27 ==
  Clock : Clock
  Source : TimeBasedEntityGenerator  Distribution=Exponential  InitialSeed=54552  Mean=Mean  GenerateEntityAtSimulationStart=off
  Timed to Event Signal : TimedToEventSignal
  setAttribute : SetAttribute  AttributeName=Route|Origin|Destination|Start  AttributeFrom=Dialog|Dialog|Dialog|Signal port  AttributeValue="[3  15  12  10   0   0]|3|10|1"  AttributeTreatAsVector=0|1|1|1  EvaluatedAttributeValue="{[3  15  12  10   0   0];3;10;[]}"
      settings: InputPortMap=u3
  OUT_Commodity : PMIOPort  Port=1  Side=Right
  wires:
  Timed to Event Signal/1 -> setAttribute/1
  Clock/1 -> Timed to Event Signal/1
  connections:
  OUT_Commodity/RConn1 -- setAttribute/RConn1
  Source/RConn1 -- setAttribute/LConn1

== system Distribution_vAggregate/Customer_4/Commodity_28 ==
  Clock : Clock
  Source : TimeBasedEntityGenerator  Distribution=Exponential  InitialSeed=60986  Mean=Mean  GenerateEntityAtSimulationStart=off
  Timed to Event Signal : TimedToEventSignal
  setAttribute : SetAttribute  AttributeName=Route|Origin|Destination|Start  AttributeFrom=Dialog|Dialog|Dialog|Signal port  AttributeValue="[4  12  17   1   0   0]|4|1|1"  AttributeTreatAsVector=0|1|1|1  EvaluatedAttributeValue="{[4  12  17   1   0   0];4;1;[]}"
      settings: InputPortMap=u3
  OUT_Commodity : PMIOPort  Port=1  Side=Right
  wires:
  Timed to Event Signal/1 -> setAttribute/1
  Clock/1 -> Timed to Event Signal/1
  connections:
  OUT_Commodity/RConn1 -- setAttribute/RConn1
  Source/RConn1 -- setAttribute/LConn1

== system Distribution_vAggregate/Customer_4/Commodity_29 ==
  Clock : Clock
  Source : TimeBasedEntityGenerator  Distribution=Exponential  InitialSeed=64203  Mean=Mean  GenerateEntityAtSimulationStart=off
  Timed to Event Signal : TimedToEventSignal
  setAttribute : SetAttribute  AttributeName=Route|Origin|Destination|Start  AttributeFrom=Dialog|Dialog|Dialog|Signal port  AttributeValue="[4  12  15   2   0   0]|4|2|1"  AttributeTreatAsVector=0|1|1|1  EvaluatedAttributeValue="{[4  12  15   2   0   0];4;2;[]}"
      settings: InputPortMap=u3
  OUT_Commodity : PMIOPort  Port=1  Side=Right
  wires:
  Timed to Event Signal/1 -> setAttribute/1
  Clock/1 -> Timed to Event Signal/1
  connections:
  OUT_Commodity/RConn1 -- setAttribute/RConn1
  Source/RConn1 -- setAttribute/LConn1

== system Distribution_vAggregate/Customer_4/Commodity_30 ==
  Clock : Clock
  Source : TimeBasedEntityGenerator  Distribution=Exponential  InitialSeed=1884  Mean=Mean  GenerateEntityAtSimulationStart=off
  Timed to Event Signal : TimedToEventSignal
  setAttribute : SetAttribute  AttributeName=Route|Origin|Destination|Start  AttributeFrom=Dialog|Dialog|Dialog|Signal port  AttributeValue="[4  12  15   3   0   0]|4|3|1"  AttributeTreatAsVector=0|1|1|1  EvaluatedAttributeValue="{[4  12  15   3   0   0];4;3;[]}"
      settings: InputPortMap=u3
  OUT_Commodity : PMIOPort  Port=1  Side=Right
  wires:
  Timed to Event Signal/1 -> setAttribute/1
  Clock/1 -> Timed to Event Signal/1
  connections:
  OUT_Commodity/RConn1 -- setAttribute/RConn1
  Source/RConn1 -- setAttribute/LConn1

== system Distribution_vAggregate/Customer_4/Commodity_31 ==
  Clock : Clock
  Source : TimeBasedEntityGenerator  Distribution=Exponential  InitialSeed=5101  Mean=Mean  GenerateEntityAtSimulationStart=off
  Timed to Event Signal : TimedToEventSignal
  setAttribute : SetAttribute  AttributeName=Route|Origin|Destination|Start  AttributeFrom=Dialog|Dialog|Dialog|Signal port  AttributeValue="[4  12   5   0   0   0]|4|5|1"  AttributeTreatAsVector=0|1|1|1  EvaluatedAttributeValue="{[4  12   5   0   0   0];4;5;[]}"
      settings: InputPortMap=u3
  OUT_Commodity : PMIOPort  Port=1  Side=Right
  wires:
  Timed to Event Signal/1 -> setAttribute/1
  Clock/1 -> Timed to Event Signal/1
  connections:
  OUT_Commodity/RConn1 -- setAttribute/RConn1
  Source/RConn1 -- setAttribute/LConn1

== system Distribution_vAggregate/Customer_4/Commodity_32 ==
  Clock : Clock
  Source : TimeBasedEntityGenerator  Distribution=Exponential  InitialSeed=8318  Mean=Mean  GenerateEntityAtSimulationStart=off
  Timed to Event Signal : TimedToEventSignal
  setAttribute : SetAttribute  AttributeName=Route|Origin|Destination|Start  AttributeFrom=Dialog|Dialog|Dialog|Signal port  AttributeValue="[4  12   6   0   0   0]|4|6|1"  AttributeTreatAsVector=0|1|1|1  EvaluatedAttributeValue="{[4  12   6   0   0   0];4;6;[]}"
      settings: InputPortMap=u3
  OUT_Commodity : PMIOPort  Port=1  Side=Right
  wires:
  Timed to Event Signal/1 -> setAttribute/1
  Clock/1 -> Timed to Event Signal/1
  connections:
  OUT_Commodity/RConn1 -- setAttribute/RConn1
  Source/RConn1 -- setAttribute/LConn1

== system Distribution_vAggregate/Customer_4/Commodity_33 ==
  Clock : Clock
  Source : TimeBasedEntityGenerator  Distribution=Exponential  InitialSeed=11535  Mean=Mean  GenerateEntityAtSimulationStart=off
  Timed to Event Signal : TimedToEventSignal
  setAttribute : SetAttribute  AttributeName=Route|Origin|Destination|Start  AttributeFrom=Dialog|Dialog|Dialog|Signal port  AttributeValue="[4  12   7   0   0   0]|4|7|1"  AttributeTreatAsVector=0|1|1|1  EvaluatedAttributeValue="{[4  12   7   0   0   0];4;7;[]}"
      settings: InputPortMap=u3
  OUT_Commodity : PMIOPort  Port=1  Side=Right
  wires:
  Timed to Event Signal/1 -> setAttribute/1
  Clock/1 -> Timed to Event Signal/1
  connections:
  OUT_Commodity/RConn1 -- setAttribute/RConn1
  Source/RConn1 -- setAttribute/LConn1

== system Distribution_vAggregate/Customer_4/Commodity_34 ==
  Clock : Clock
  Source : TimeBasedEntityGenerator  Distribution=Exponential  InitialSeed=14752  Mean=Mean  GenerateEntityAtSimulationStart=off
  Timed to Event Signal : TimedToEventSignal
  setAttribute : SetAttribute  AttributeName=Route|Origin|Destination|Start  AttributeFrom=Dialog|Dialog|Dialog|Signal port  AttributeValue="[4  12  15   8   0   0]|4|8|1"  AttributeTreatAsVector=0|1|1|1  EvaluatedAttributeValue="{[4  12  15   8   0   0];4;8;[]}"
      settings: InputPortMap=u3
  OUT_Commodity : PMIOPort  Port=1  Side=Right
  wires:
  Timed to Event Signal/1 -> setAttribute/1
  Clock/1 -> Timed to Event Signal/1
  connections:
  OUT_Commodity/RConn1 -- setAttribute/RConn1
  Source/RConn1 -- setAttribute/LConn1

== system Distribution_vAggregate/Customer_4/Commodity_35 ==
  Clock : Clock
  Source : TimeBasedEntityGenerator  Distribution=Exponential  InitialSeed=17969  Mean=Mean  GenerateEntityAtSimulationStart=off
  Timed to Event Signal : TimedToEventSignal
  setAttribute : SetAttribute  AttributeName=Route|Origin|Destination|Start  AttributeFrom=Dialog|Dialog|Dialog|Signal port  AttributeValue="[4  12  15   9   0   0]|4|9|1"  AttributeTreatAsVector=0|1|1|1  EvaluatedAttributeValue="{[4  12  15   9   0   0];4;9;[]}"
      settings: InputPortMap=u3
  OUT_Commodity : PMIOPort  Port=1  Side=Right
  wires:
  Timed to Event Signal/1 -> setAttribute/1
  Clock/1 -> Timed to Event Signal/1
  connections:
  OUT_Commodity/RConn1 -- setAttribute/RConn1
  Source/RConn1 -- setAttribute/LConn1

== system Distribution_vAggregate/Customer_4/Commodity_36 ==
  Clock : Clock
  Source : TimeBasedEntityGenerator  Distribution=Exponential  InitialSeed=21186  Mean=Mean  GenerateEntityAtSimulationStart=off
  Timed to Event Signal : TimedToEventSignal
  setAttribute : SetAttribute  AttributeName=Route|Origin|Destination|Start  AttributeFrom=Dialog|Dialog|Dialog|Signal port  AttributeValue="[4  12  10   0   0   0]|4|10|1"  AttributeTreatAsVector=0|1|1|1  EvaluatedAttributeValue="{[4  12  10   0   0   0];4;10;[]}"
      settings: InputPortMap=u3
  OUT_Commodity : PMIOPort  Port=1  Side=Right
  wires:
  Timed to Event Signal/1 -> setAttribute/1
  Clock/1 -> Timed to Event Signal/1
  connections:
  OUT_Commodity/RConn1 -- setAttribute/RConn1
  Source/RConn1 -- setAttribute/LConn1

== system Distribution_vAggregate/Customer_5/Commodity_37 ==
  Clock : Clock
  Source : TimeBasedEntityGenerator  Distribution=Exponential  InitialSeed=24403  Mean=Mean  GenerateEntityAtSimulationStart=off
  Timed to Event Signal : TimedToEventSignal
  setAttribute : SetAttribute  AttributeName=Route|Origin|Destination|Start  AttributeFrom=Dialog|Dialog|Dialog|Signal port  AttributeValue="[5  12  17   1   0   0]|5|1|1"  AttributeTreatAsVector=0|1|1|1  EvaluatedAttributeValue="{[5  12  17   1   0   0];5;1;[]}"
      settings: InputPortMap=u3
  OUT_Commodity : PMIOPort  Port=1  Side=Right
  wires:
  Timed to Event Signal/1 -> setAttribute/1
  Clock/1 -> Timed to Event Signal/1
  connections:
  OUT_Commodity/RConn1 -- setAttribute/RConn1
  Source/RConn1 -- setAttribute/LConn1

== system Distribution_vAggregate/Customer_5/Commodity_38 ==
  Clock : Clock
  Source : TimeBasedEntityGenerator  Distribution=Exponential  InitialSeed=27620  Mean=Mean  GenerateEntityAtSimulationStart=off
  Timed to Event Signal : TimedToEventSignal
  setAttribute : SetAttribute  AttributeName=Route|Origin|Destination|Start  AttributeFrom=Dialog|Dialog|Dialog|Signal port  AttributeValue="[5  12  15   2   0   0]|5|2|1"  AttributeTreatAsVector=0|1|1|1  EvaluatedAttributeValue="{[5  12  15   2   0   0];5;2;[]}"
      settings: InputPortMap=u3
  OUT_Commodity : PMIOPort  Port=1  Side=Right
  wires:
  Timed to Event Signal/1 -> setAttribute/1
  Clock/1 -> Timed to Event Signal/1
  connections:
  OUT_Commodity/RConn1 -- setAttribute/RConn1
  Source/RConn1 -- setAttribute/LConn1
